simulink model "Aula1"  (R2021b)
settings: Solver=VariableStepAuto  StartTime=0.0  StopTime=100  MaxStep=1  RelTol=1e-3
undefined symbols (not defined in the file): beta, I0, r, R0, S0
settings Model: Creator=20.01305-0  LastModifiedBy=20.01305-0

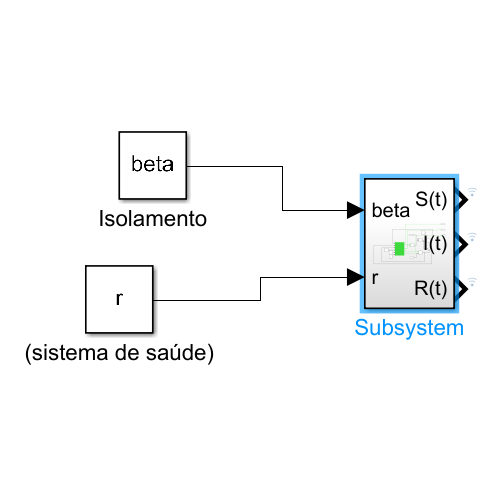
[thumbnail: Simulink's stored preview of the top-level diagram]
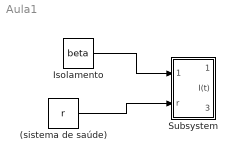
== system Aula1 ==
  (sistema de saúde) : Constant  Value=r
  Isolamento : Constant  Value=beta  SampleTime=beta
  Subsystem : Subsystem
  wires:
  Isolamento/1 -> Subsystem/1(beta)
  (sistema de saúde)/1 -> Subsystem/2(r)

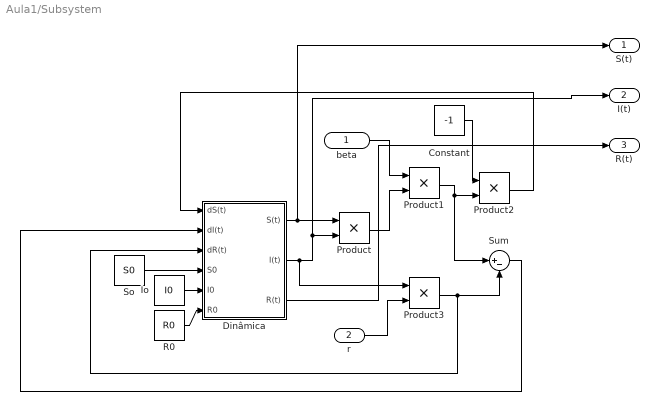
== system Aula1/Subsystem ==
  beta : Inport
  r : Inport  Port=2
  Constant : Constant  Value=-1
  Dinâmica : Subsystem
  Io : Constant  Value=I0
  Product{,1..3} (4 alike) : Product
  R0 : Constant  Value=R0
  So : Constant  Value=S0  SampleTime=S0
  Sum : Sum  Inputs=|+-
  S(t) : Outport
  I(t) : Outport  Port=2
  R(t) : Outport  Port=3
  wires:
  Io/1 -> Dinâmica/5(I0)
  Dinâmica/3(R(t)) -> R(t)/1
  So/1 -> Dinâmica/4(S0)
  Sum/1 -> Dinâmica/2(dI(t))
  Product/1 -> Product1/2
  R0/1 -> Dinâmica/6(R0)
  Product3/1 -> Dinâmica/3(dR(t)), Sum/2
  Product2/1 -> Dinâmica/1(dS(t))
  beta/1 -> Product1/1
  Constant/1 -> Product2/1
  Product1/1 -> Sum/1, Product2/2
  r/1 -> Product3/2
  Dinâmica/1(S(t)) -> S(t)/1, Product/1
  Dinâmica/2(I(t)) -> Product3/1, I(t)/1, Product/2

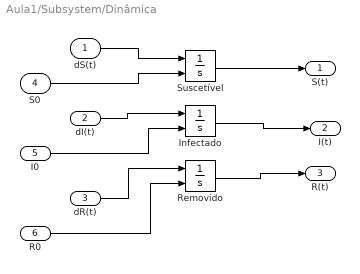
== system Aula1/Subsystem/Dinâmica ==
  dS(t) : Inport
  dI(t) : Inport  Port=2
  dR(t) : Inport  Port=3
  S0 : Inport  Port=4
  I0 : Inport  Port=5
  R0 : Inport  Port=6
  Infectado : Integrator  InitialConditionSource=external
  Removido : Integrator  InitialConditionSource=external
  Suscetível : Integrator  InitialConditionSource=external
  S(t) : Outport
  I(t) : Outport  Port=2
  R(t) : Outport  Port=3
  wires:
  Removido/1 -> R(t)/1
  S0/1 -> Suscetível/2
  dS(t)/1 -> Suscetível/1
  I0/1 -> Infectado/2
  R0/1 -> Removido/2
  Suscetível/1 -> S(t)/1
  dI(t)/1 -> Infectado/1
  dR(t)/1 -> Removido/1
  Infectado/1 -> I(t)/1
